simulink model "lqrpilot"  (R2025a)
settings: Solver=ode45  StartTime=0.0  StopTime=60  RelTol=1e-3  EnableMultiTasking=on
PreLoadFcn:
  | load lqrpilotData
values from neighbouring files (symbols this model uses):
  B = double(B)    [Copy_of_InvertedPendulum_Equations.m]    (also in Gemini_trial.m = double(subs(B_sym, params, values)); Gemini_trial_v2.m = double(subs(B_sym, params, values)); run_pendcart.m = [0; 1/M; 0; b*1/(M*L)]; untitled5.m = double(subs(B_sym, params, values)))
undefined symbols (not defined in the file or in its folder): A15, K_lqr
settings Model: Creator=The MathWorks, Inc.  LastModifiedBy=omarfahmy
settings SolverCC: AlgebraicLoopSolver=TrustRegion
settings DataIOCC: LimitDataPoints=on  SaveFormat=Array  ReturnWorkspaceOutputs=off
settings OptimizationCC: BlockReduction=off  BooleanDataType=off  ReuseModelBlockBuffer=off  ExpressionDepthLimit=2147483647.0  LifeSpan=inf
settings DebuggingCC: AlgebraicLoopMsg=none  SaveWithParameterizedLinksMsg=none  UnderspecifiedInitializationDetection=Classic  MergeDetectMultiDrivingBlocksExec=none  SignalResolutionControl=TryResolveAllWithWarning  MultiTaskDSMMsg=warning  MultiTaskCondExecSysMsg=none  FcnCallInpInsideContextMsg=warning  UnconnectedInputMsg=warning  UnconnectedOutputMsg=warning  UnconnectedLineMsg=warning  StateNameClashWarn=warning  SFUnexpectedBacktrackingDiag=warning  SFNoUnconditionalDefaultTransitionDiag=warning  SFExecutionAtInitializationDiag=none  ArithmeticOperatorsInVariantConditions=warning
settings HardwareCC: ProdBitPerPointer=32.0  ProdBitPerSizeT=32.0  ProdBitPerPtrDiffT=32.0  ProdLargestAtomicFloat=None  ProdIntDivRoundTo=Undefined  ProdEndianess=Unspecified  ProdWordSize=32.0  ProdHWDeviceType=32-bit Generic  TargetUnknown=on
settings ModelReferenceCC: PropagateSignalLabelsOutOfModel=off
settings SFSimCC: SimUseLocalCustomCode=off  CustomCodeUndefinedFunction=UseInterfaceOnly
settings RTWCC: RTWUseLocalCustomCode=off  GPUComputeCapability=3.5
settings CodeAppCC: StateflowObjectComments=on
settings GRTTargetCC: TargetLangStandard=C89/C90 (ANSI)  CombineOutputUpdateFcns=off  GRTInterface=on
settings ConfigComp: CovMetricSettings=dw  CovSaveCumulativeToWorkspaceVar=on  CovSaveSingleToWorkspaceVar=on

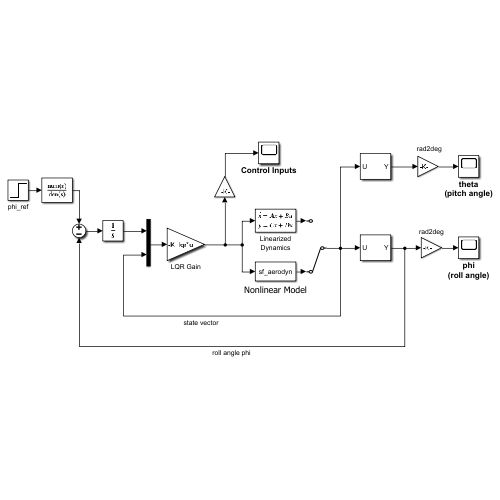
[thumbnail: Simulink's stored preview of the top-level diagram]
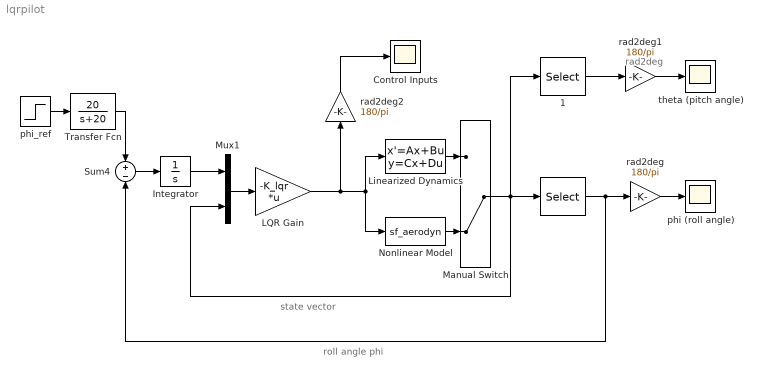
== system lqrpilot ==
  note: state vector
  note: roll angle phi
  note: rad2deg
  " " : Selector  InputPortWidth=8  IndexOptions=Index vector (dialog)  Indices=8  OutputSizes=1
  " 1" : Selector  InputPortWidth=8  IndexOptions=Index vector (dialog)  Indices=7  OutputSizes=1
  Control Inputs : Scope
      settings: TimeSpan=60  ActiveDisplayYMinimum=-30  ActiveDisplayYMaximum=15  DataLoggingVariableName=ScopeData2
  Integrator : Integrator
  LQR Gain : Gain  Gain=-K_lqr  Multiplication=Matrix(K*u)  SaturateOnIntegerOverflow=on  OutDataTypeStr=Inherit: Same as input  ParamDataTypeStr=Inherit: Same as input
  Linearized Dynamics : StateSpace  A=A15  B=B  C=eye(8)  D=zeros(8,4)  InitialCondition=0
  Manual Switch : ManualSwitch  CurrentSetting=0
  Mux1 : Mux  Inputs=2
  Nonlinear Model : M-S-Function  FunctionName=sf_aerodyn
  Sum4 : Sum  Inputs=+-  InputSameDT=on  SaturateOnIntegerOverflow=on  OutDataTypeStr=Inherit: Same as first input
  Transfer Fcn : TransferFcn  Numerator=20  Denominator=[1 20]
  phi (roll angle) : Scope
      settings: TimeSpan=60  ActiveDisplayYMinimum=-20  ActiveDisplayYMaximum=60
  phi_ref : Step  Time=0  After=pi/3  SampleTime=0
  rad2deg : Gain  Gain=180/pi  SaturateOnIntegerOverflow=on  OutDataTypeStr=Inherit: Same as input  ParamDataTypeStr=Inherit: Same as input
  rad2deg1 : Gain  Gain=180/pi  SaturateOnIntegerOverflow=on  OutDataTypeStr=Inherit: Same as input  ParamDataTypeStr=Inherit: Same as input
  rad2deg2 : Gain  Gain=180/pi  SaturateOnIntegerOverflow=on  OutDataTypeStr=Inherit: Same as input  ParamDataTypeStr=Inherit: Same as input
  theta (pitch angle) : Scope
      settings: TimeSpan=60  ActiveDisplayYMinimum=-7.5
  wires:
  phi_ref/1 -> Transfer Fcn/1
  Sum4/1 -> Integrator/1
  Mux1/1 -> LQR Gain/1
  Integrator/1 -> Mux1/1
  Transfer Fcn/1 -> Sum4/1
  LQR Gain/1 -> Nonlinear Model/1, Linearized Dynamics/1, rad2deg2/1
  Linearized Dynamics/1 -> Manual Switch/1
  Nonlinear Model/1 -> Manual Switch/2
  rad2deg/1 -> phi (roll angle)/1
  " 1"/1 -> rad2deg1/1
  rad2deg1/1 -> theta (pitch angle)/1
  rad2deg2/1 -> Control Inputs/1
  Manual Switch/1 -> " "/1, " 1"/1, Mux1/2
  " "/1 -> rad2deg/1, Sum4/2
